simulink model "sigma_delta_cosim"  (Simulink 7.7)
settings: Solver=FixedStepDiscrete  SolverMode=SingleTasking  StartTime=0.0  StopTime=.01  FixedStep=1e-7  RelTol=1e-3
undefined symbols (not defined in the file or in its folder): dfilt, fdesignblkfcn, gcbh
libraries: modelsimlib x1, dsparch4 x1
settings Model: Creator=embed  LastModifiedBy=embed

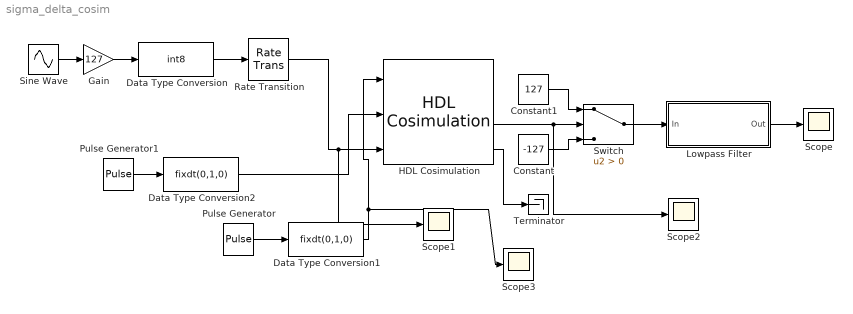
== system sigma_delta_cosim ==
  Constant : Constant  Value=-127
  Constant1 : Constant  Value=127
  Data Type Conversion : DataTypeConversion  OutDataTypeStr=int8
  Data Type Conversion1 : DataTypeConversion  OutDataTypeStr=fixdt(0,1,0)
  Data Type Conversion2 : DataTypeConversion  OutDataTypeStr=fixdt(0,1,0)
  Gain : Gain  Gain=127
  HDL Cosimulation : modelsimlib/HDL Cosimulation  SystemSampleTime=-1  PortPaths=/usbif/clk;/usbif/clk_out;/usbif/ctl0;/usbif/data_in;/usbif/data_out;/usbif/pwm_out;/usbif/rdy  PortModes=[1 2 1 1 2 2 2 ]  PortTimes=[-1,1e-7,-1,-1,1e-7,1e-7,1e-7]  PortSigns=[-1 -1 -1 -1 0 0 0 ]  PortFracLengths=[0,0,0,0,0,0,0]  CommLocal=on  CommSharedMemory=off  CommPortNumber=4449  CommShowInfo=on  ClockModes=[]  ClockTimes=[]  TclPreSimCommand="puts \"Running Simulink Cosimulation block.\""  TclPostSimCommand="puts \"done\""  TimingMode=Tick  TimingScaleFactor=1e7  idxCellArray={'UNUSED_VAR'}  CosimBypass=Full Simulation  AllowDirectFeedthrough=off  ProductName=EDA Simulator Link MQ  RunAutoTimescale=off  HdlClocks=0
  Lowpass Filter : Subsystem  DialogController=fdesignblkfcn  DialogControllerArgs=DataTag1  InitFcn=fdesignblkfcn(gcbh, {'InitFcn'});
      settings: CopyFcn=fdesignblkfcn(gcbh, {'CopyFcn'});
      mask Type: Lowpass Filter
      mask Description: Design a lowpass filter
      mask Help: helpview(mapfilelocation('dsp'), 'dsplowpassfilter');
      mask Display: disp('Lowpass')
  Pulse Generator : DiscretePulseGenerator  SampleTime=1e-7
  Pulse Generator1 : DiscretePulseGenerator  SampleTime=512/10e6
  Rate Transition : RateTransition  OutPortSampleTime=1e-7
  Scope{,1..3} (4 alike) : Scope
      Scope settings: YMin=-150  YMax=150  MaxDataPoints=100000
      Scope1 settings: YMin=-150  YMax=150  MaxDataPoints=100000
      Scope2 settings: YMin=-150  YMax=150  SaveName=ScopeData2  MaxDataPoints=100000
      Scope3 settings: YMin=-150  YMax=150  SaveName=ScopeData3  MaxDataPoints=100000
  Sine Wave : Sin  SineType=Sample based  Samples=195  SampleTime=512/10e6
  Switch : Switch  Criteria=u2 > Threshold  OutDataTypeStr=Inherit: Inherit via back propagation
  Terminator : Terminator
  wires:
  Sine Wave/1 -> Gain/1
  Gain/1 -> Data Type Conversion/1
  Data Type Conversion/1 -> Rate Transition/1
  Constant1/1 -> Switch/1
  Constant/1 -> Switch/3
  Switch/1 -> Lowpass Filter/1(In)
  Lowpass Filter/1(Out) -> Scope/1
  Rate Transition/1 -> HDL Cosimulation/3, Scope1/1
  HDL Cosimulation/4 -> Terminator/1
  Pulse Generator/1 -> Data Type Conversion1/1
  Data Type Conversion1/1 -> HDL Cosimulation/1, Scope3/1
  Pulse Generator1/1 -> Data Type Conversion2/1
  Data Type Conversion2/1 -> HDL Cosimulation/2
  HDL Cosimulation/3 -> Switch/2, Scope2/1

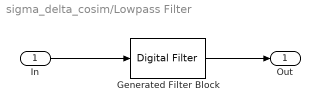
== system sigma_delta_cosim/Lowpass Filter ==
  In : Inport
  Generated Filter Block : dsparch4/Digital Filter  Tag=BlockMethodSubSystem  TypePopup=FIR (all zeros)  IIRFiltStruct=Direct form II transposed  AllPoleFiltStruct=Direct form  FIRFiltStruct=Direct form  CoeffSource=Specify via dialog  NumCoeffs=[-0.00118476584785469 -0.000130803156680574 -0.000137422068460495 -0.000143919079247468 -0.000150129111891543 -0.000156142406914831 -0.000161808864671033 -0.000167117858059886 -0.000171994954768621 -0.000176432916968601 -0.000180295015102807 -0.000183601447425357 -0.000186244588772191 -0.00018820407653106 -0.000189397546922163 -0.000189815179967878 -0.000189378565185153 -0.000188086844117713 -0.000185878675385287 -0.000182705681898147 -0.000178520470550318 -0.000173211791368695 -0.000166691526574751 -0.000158801072461655 -0.000149477855082444 -0.000138504644208159 -0.000126056570800368 -0.000112041581679819 -9.69167234137775e-005 -8.0459960834572e-005 -6.28502050373026e-005 -3.99668572469413e-005 -1.85475382492662e-005 5.69319240332647e-006 3.23861249849271e-005 6.06428726127771e-005 9.14023309533662e-005 0.000124078364735737 0.000159205831433732 0.000196418401982276 0.000236187494852051 0.000278143977520299 0.000322722434938506 0.000369653981943196 0.000419300792648991 0.000471418413607005 0.000526336665716825 0.000583800858877049 0.000644107713567938 0.000707016499247755 0.000772770423509413 0.000841180342106741 0.00091251222503524 0.000986608134069558 0.00106373413973953 0.00114372036019421 0.00122664937226443 0.00131231999922691 0.00140080857517382 0.00149210604629858 0.00158650990830528 0.00168413923021004 0.00178374767545044 0.00188666100582717 0.00199250493472929 0.0021007208108203 0.00221205293149999 0.00232580542586945 0.00244240619331815 0.00256144264480469 0.00268320066647761 0.00280721991780864 0.0029338371548847 0.00306264069522413 0.00319388049089356 0.00332717706000522 0.00346276314134365 0.00360024664805553 0.00373983927115151 0.00388112393714378 0.00402426829384525 0.00416890853532495 0.00431522658579233 0.00446286852678186 0.0046120062135098 0.00476222652953532 0.0049136006585844 0.00506577167721975 0.00521886206182787 0.0053725992270446 0.00552710267571209 0.00568189889211809 0.00583679822071849 0.00599206733616528 0.00614734761318997 0.00630219211597086 0.00645711021795362 0.00661126954310569 0.00676505204353828 0.00691795374536605 0.00707007513344941 0.00722094451138691 0.0073707941909542 0.00751909980538466 0.00766602338410489 0.00781111733632051 0.00795454325618579 0.00809584510682575 0.00823516873386113 0.00837202553171585 0.00850656850242501 0.0086383799940291 0.00876761785195569 0.00889386081823082 0.0090172489151635 0.00913730860284804 0.00925417775544187 0.00936747794112871 0.00947737824922211 0.00958351090159572 0.0096859948880864 0.00978435136710049 0.00987876721716443 0.00996906828065999 0.0100551233826258 0.0101366358258843 0.0102140293489938 0.010286541162993 0.0103546987371931 0.0104180145361652 0.0104766046304591 0.010530231366637 0.0105791285372569 0.0106228576037114 0.0106616942885663 0.0106953253686012 0.0107240066212253 0.0107474004217175 0.01076575051574 0.0107787120463055 0.010786599333258 0.0107891299534653 0.010786599333258 0.0107787120463055 0.01076575051574 0.0107474004217175 0.0107240066212253 0.0106953253686012 0.0106616942885663 0.0106228576037114 0.0105791285372569 0.010530231366637 0.0104766046304591 0.0104180145361652 0.0103546987371931 0.010286541162993 0.0102140293489938 0.0101366358258843 0.0100551233826258 0.00996906828065999 0.00987876721716443 0.00978435136710049 0.0096859948880864 0.00958351090159572 0.00947737824922211 0.00936747794112871 0.00925417775544187 0.00913730860284804 0.0090172489151635 0.00889386081823082 0.00876761785195569 0.0086383799940291 0.00850656850242501 0.00837202553171585 0.00823516873386113 0.00809584510682575 0.00795454325618579 0.00781111733632051 0.00766602338410489 0.00751909980538466 0.0073707941909542 0.00722094451138691 0.00707007513344941 0.00691795374536605 0.00676505204353828 0.00661126954310569 0.00645711021795362 0.00630219211597086 0.00614734761318997 0.00599206733616528 0.00583679822071849 0.00568189889211809 0.00552710267571209 0.0053725992270446 0.00521886206182787 0.00506577167721975 0.0049136006585844 0.00476222652953532 ...(+1789 chars)]  DenCoeffs=[1 0.1]  BiQuadCoeffs=[1 0.3 0.4 1 0.1 0.2]  LatticeCoeffs=[0.2 0.4]  denIgnore=on  FiltPerSampPopup=One filter per frame  IC=0  ICnum=0  ICden=0  roundingMode=Floor  overflowMode=off  ScaleValues=1  scaleValueFracLength=14  stageInFracLength=15  stageOutFracLength=15  FilterSource=Specify via dialog  dfiltObjectName=dfilt.dffir([1 2 1])  InputProcessing=Columns as channels (frame based)
  Out : Outport
  wires:
  In/1 -> Generated Filter Block/1
  Generated Filter Block/1 -> Out/1
